simulink model "Cooperative_Quad_Rev01_4Agents_9"  (R2017b)
settings: Solver=ode45  StartTime=0.0  StopTime=120  RelTol=1e-3  EnableMultiTasking=on
InitFcn:
  | constant_Rev01_4Agents_9
values from neighbouring files (symbols this model uses):
  alpha = 0.1    [constant_Rev01_4Agents_9.m]
  alpha1 = 0.01    [constant_Rev01_4Agents_9.m]
  AN = [     0 1 0 0 ... (first row only)    [constant_Rev01_4Agents_9.m]
  B = 1e0*eye(n)    [constant_Rev01_4Agents_9.m]
  BBT_inv = ((B'*B)^(-1))*B'    [constant_Rev01_4Agents_9.m]
  BN = [     1 0 0 0 ... (first row only)    [constant_Rev01_4Agents_9.m]
  epsilon_struct = struct('data',epsilon_InitVal)    [constant_Rev01_4Agents_9.m]
  g = 9.81    [constant_Rev01_4Agents_9.m]
  gamma_0 = 1e+1*diag([1e-3*ones(6,1);1e-0*ones(6,1)])    [constant_Rev01_4Agents_9.m]
  gamma_1 = 1e+3*diag([1e-3*ones(6,1);1e0*ones(6,1)])    [constant_Rev01_4Agents_9.m]
  H = L + BN    [constant_Rev01_4Agents_9.m]
  J = 1.2416e-3 * diag([1 1 2],0)    [constant_Rev01_4Agents_9.m]
  k1 = 1    [constant_Rev01_4Agents_9.m]
  k2 = 1    [constant_Rev01_4Agents_9.m]
  Ka = 0.01    [constant_Rev01_4Agents_9.m]
  Kd = 0.01    [constant_Rev01_4Agents_9.m]
  Kf = 1e-5    (= 1e-05)    [constant_Rev01_4Agents_9.m]
  Ki = 1    [constant_Rev01_4Agents_9.m]
  Kt = 0.01 * Kf    (= 1e-07)    [constant_Rev01_4Agents_9.m]
  Lq = 0.2    [constant_Rev01_4Agents_9.m]
  M = 2    [constant_Rev01_4Agents_9.m]
  n = 12    [constant_Rev01_4Agents_9.m]
  N = 4    [constant_Rev01_4Agents_9.m]
  n0 = 3    [constant_Rev01_4Agents_9.m]
  Observer_Gain = 100    [constant_Rev01_4Agents_9.m]
  Observer_Gain1 = 10    [constant_Rev01_4Agents_9.m]
  Q = 1e-3*eye(n)    [constant_Rev01_4Agents_9.m]
  R = 1e-0*eye(n)    [constant_Rev01_4Agents_9.m]
  rho_0 = 1e+1    (= 10)    [constant_Rev01_4Agents_9.m]
  rho_1 = 1e-1    (= 0.1)    [constant_Rev01_4Agents_9.m]
  RM_1 = RM^(-1)    [constant_Rev01_4Agents_9.m]
  T_struct = struct('data',T_InitVal)    [constant_Rev01_4Agents_9.m]
  U_dot0_M = U_dot0_m*ones(n0,1)    [constant_Rev01_4Agents_9.m]
  Upsilon_M = Upsilon_m*ones(n0,1)    [constant_Rev01_4Agents_9.m]
undefined symbols (not defined in the file or in its folder): sigbuilder_block
(part 1 of 2)
settings Model: SimulationMode=rapid-accelerator  Creator=hp  LastModifiedBy=ali.safaei
settings DataIOCC: LimitDataPoints=on  SaveFormat=Array
settings OptimizationCC: LifeSpan=inf
settings DebuggingCC: UnderspecifiedInitializationDetection=Classic  MergeDetectMultiDrivingBlocksExec=none  SFUnexpectedBacktrackingDiag=warning  SFNoUnconditionalDefaultTransitionDiag=warning  SFExecutionAtInitializationDiag=none
settings HardwareCC: ProdBitPerPointer=32  ProdBitPerSizeT=32  ProdBitPerPtrDiffT=32  ProdLargestAtomicFloat=None  ProdIntDivRoundTo=Undefined  ProdEndianess=Unspecified  ProdWordSize=32  ProdHWDeviceType=32-bit Generic
settings ModelReferenceCC: PropagateSignalLabelsOutOfModel=off
settings CodeAppCC: StateflowObjectComments=on
settings GRTTargetCC: TargetLangStandard=C89/C90 (ANSI)  GeneratePreprocessorConditionals=Disable all
settings ConfigComp: CovMetricSettings=dw  CovHtmlReporting=on  CovSaveCumulativeToWorkspaceVar=on  CovSaveSingleToWorkspaceVar=on  CovExternalEMLEnable=off

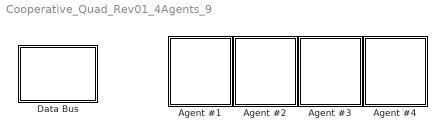
== system Cooperative_Quad_Rev01_4Agents_9 ==
  Agent #1 : Subsystem
  Agent #2 : Subsystem
  Agent #3 : Subsystem
  Agent #4 : Subsystem
  "Data Bus " : Subsystem

== system Cooperative_Quad_Rev01_4Agents_9/Agent #1 ==
  Agent # : Constant
  Controller interpreter : MATLAB Function  TreatAsAtomicUnit=on
  Decenteralized Cooperaive Controller #1 : Subsystem
  Plant #1 : Subsystem
  tag scope: x1=global
  wires:
  Decenteralized Cooperaive Controller #1/1(u1) -> Controller interpreter/1(U)
  Agent #/1 -> Decenteralized Cooperaive Controller #1/1(Agent #)
  Plant #1/1(X) -> [x1]
  Controller interpreter/1(u) -> Plant #1/1(U)

== system Cooperative_Quad_Rev01_4Agents_9/Agent #2 ==
  Agent # : Constant  Value=2
  Controller interpreter : MATLAB Function  TreatAsAtomicUnit=on
  Decenteralized Cooperaive Controller #2 : Subsystem
  Plant #2 : Subsystem
  tag scope: x2=global
  wires:
  Controller interpreter/1(u) -> Plant #2/1(U)
  Plant #2/1(X) -> [x2]
  Agent #/1 -> Decenteralized Cooperaive Controller #2/1(Agent #)
  Decenteralized Cooperaive Controller #2/1(u2) -> Controller interpreter/1(U)

== system Cooperative_Quad_Rev01_4Agents_9/Agent #3 ==
  Agent # : Constant  Value=3
  Controller interpreter : MATLAB Function  TreatAsAtomicUnit=on
  Decenteralized Cooperaive Controller #3 : Subsystem
  Plant #3 : Subsystem
  tag scope: x3=global
  wires:
  Decenteralized Cooperaive Controller #3/1(u3) -> Controller interpreter/1(U)
  Agent #/1 -> Decenteralized Cooperaive Controller #3/1(Agent #)
  Plant #3/1(X) -> [x3]
  Controller interpreter/1(u) -> Plant #3/1(U)

== system Cooperative_Quad_Rev01_4Agents_9/Agent #4 ==
  Agent # : Constant  Value=4
  Controller interpreter : MATLAB Function  TreatAsAtomicUnit=on
  Decenteralized Cooperaive Controller #4 : Subsystem
  Plant #4 : Subsystem
  tag scope: x4=global
  wires:
  Controller interpreter/1(u) -> Plant #4/1(U)
  Plant #4/1(X) -> [x4]
  Agent #/1 -> Decenteralized Cooperaive Controller #4/1(Agent #)
  Decenteralized Cooperaive Controller #4/1(u4) -> Controller interpreter/1(U)

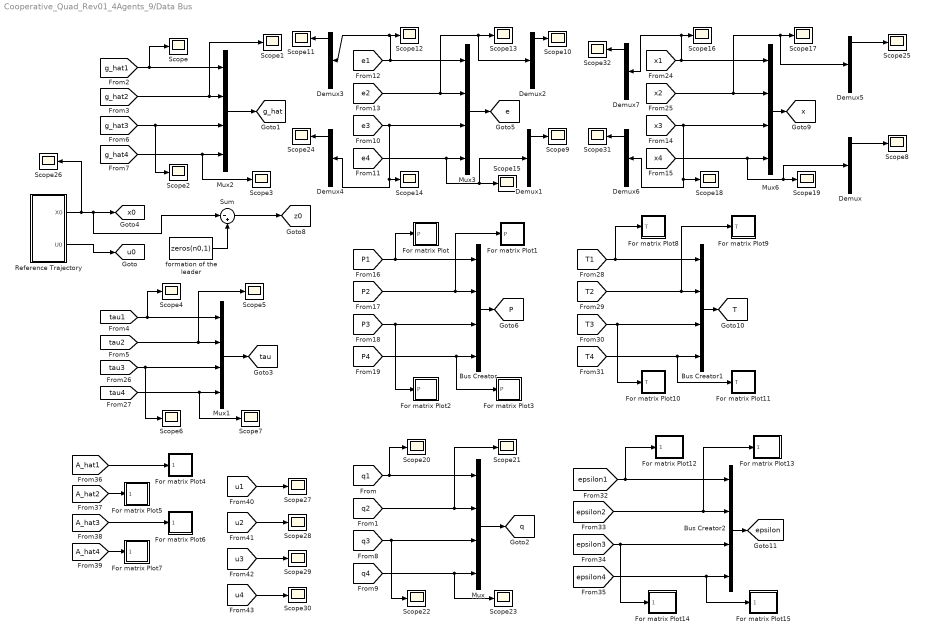
== system Cooperative_Quad_Rev01_4Agents_9/Data Bus  ==
  Bus Creator : BusCreator  Inputs=4  OutDataTypeStr=Bus: P_bus
  Bus Creator1 : BusCreator  Inputs=4  OutDataTypeStr=Bus: T_bus
  Bus Creator2 : BusCreator  Inputs=4  OutDataTypeStr=Bus: epsilon_bus
  Demux{,1..7} (8 alike) : Demux
  For matrix Plot : Subsystem
  For matrix Plot1 : Subsystem
  For matrix Plot10 : Subsystem
  For matrix Plot11 : Subsystem
  For matrix Plot12 : Subsystem
  For matrix Plot13 : Subsystem
  For matrix Plot14 : Subsystem
  For matrix Plot15 : Subsystem
  For matrix Plot2 : Subsystem
  For matrix Plot3 : Subsystem
  For matrix Plot4 : Subsystem
  For matrix Plot5 : Subsystem
  For matrix Plot6 : Subsystem
  For matrix Plot7 : Subsystem
  For matrix Plot8 : Subsystem
  For matrix Plot9 : Subsystem
  Mux{,1..3,6} (5 alike) : Mux
  Reference Trajectory : Subsystem
  Scope{,1..32} (33 alike) : Scope
  Sum : Sum  Inputs=|-+
  formation of the leader : Constant  Value=zeros(n0,1)
  tag scope: P=global, T=global, e=global, epsilon=global, g_hat=global, q=global, tau=global, u0=global, x0=global, x=global, z0=global
  wires:
  [q2] -> Scope21/1, Mux/2
  [tau1] -> Scope4/1, Mux1/1
  [tau2] -> Scope5/1, Mux1/2
  Mux1/1 -> [tau]
  [q1] -> Scope20/1, Mux/1
  Reference Trajectory/2(U0) -> [u0]
  [g_hat2] -> Mux2/2, Scope1/1
  Mux2/1 -> [g_hat]
  [g_hat1] -> Mux2/1, Scope/1
  Mux/1 -> [q]
  Reference Trajectory/1(X0) -> [x0], Sum/1, Scope26/1
  [e2] -> Demux2/1, Scope13/1, Mux3/2
  [e1] -> Scope12/1, Demux3/1, Mux3/1
  Mux3/1 -> [e]
  [P2] -> For matrix Plot1/1(P), Bus Creator/2
  [P1] -> For matrix Plot/1(P), Bus Creator/1
  Bus Creator/1 -> [P]
  Sum/1 -> [z0]
  formation of the leader/1 -> Sum/2
  [x1] -> Scope16/1, Demux7/1, Mux6/1
  Mux6/1 -> [x]
  [g_hat3] -> Scope2/1, Mux2/3
  [g_hat4] -> Scope3/1, Mux2/4
  [q4] -> Scope23/1, Mux/4
  [q3] -> Scope22/1, Mux/3
  [e3] -> Demux4/1, Scope14/1, Mux3/3
  [e4] -> Demux1/1, Scope15/1, Mux3/4
  [x3] -> Demux6/1, Scope18/1, Mux6/3
  [x4] -> Demux/1, Scope19/1, Mux6/4
  [P3] -> For matrix Plot2/1(P), Bus Creator/3
  [P4] -> For matrix Plot3/1(P), Bus Creator/4
  [tau3] -> Scope6/1, Mux1/3
  [tau4] -> Scope7/1, Mux1/4
  [T2] -> For matrix Plot9/1(T), Bus Creator1/2
  [T1] -> For matrix Plot8/1(T), Bus Creator1/1
  Bus Creator1/1 -> [T]
  [T3] -> For matrix Plot10/1(T), Bus Creator1/3
  [T4] -> For matrix Plot11/1(T), Bus Creator1/4
  [epsilon2] -> For matrix Plot13/1(epsilon), Bus Creator2/2
  [epsilon1] -> For matrix Plot12/1(epsilon), Bus Creator2/1
  Bus Creator2/1 -> [epsilon]
  [epsilon3] -> For matrix Plot14/1(epsilon), Bus Creator2/3
  [epsilon4] -> For matrix Plot15/1(epsilon), Bus Creator2/4
  [A_hat2] -> For matrix Plot5/1(A_hat)
  [A_hat1] -> For matrix Plot4/1(A_hat)
  [A_hat3] -> For matrix Plot6/1(A_hat)
  [A_hat4] -> For matrix Plot7/1(A_hat)
  [u2] -> Scope28/1
  [u1] -> Scope27/1
  [u4] -> Scope30/1
  [u3] -> Scope29/1
  Demux/1 -> Scope8/1
  Demux1/1 -> Scope9/1
  Demux2/1 -> Scope10/1
  Demux3/1 -> Scope11/1
  Demux4/1 -> Scope24/1
  [x2] -> Demux5/1, Scope17/1, Mux6/2
  Demux5/1 -> Scope25/1
  Demux6/1 -> Scope31/1
  Demux7/1 -> Scope32/1

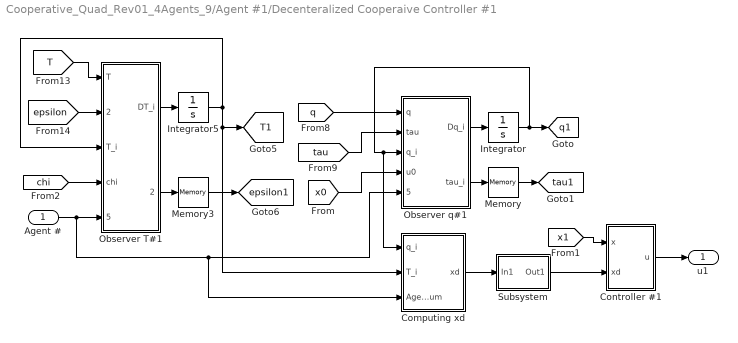
== system Cooperative_Quad_Rev01_4Agents_9/Agent #1/Decenteralized Cooperaive Controller #1 ==
  Agent # : Inport
  "Computing xd " : MATLAB Function  TreatAsAtomicUnit=on
  Controller #1 : Subsystem
  Integrator : Integrator  InitialCondition=zeros(n0,1)
  Integrator5 : Integrator  InitialCondition=zeros(N+1,n0)
  Memory : Memory  InitialCondition=zeros(n0,1)
  Memory3 : Memory  InitialCondition=zeros(N+1,n0)
  Observer T#1 : MATLAB Function  TreatAsAtomicUnit=on
  Observer q#1 : MATLAB Function  TreatAsAtomicUnit=on
  Subsystem : Subsystem
  u1 : Outport
  tag scope: T1=global, epsilon1=global, q1=global, tau1=global
  wires:
  [x0] -> Observer q#1/4(u0)
  [epsilon] -> Observer T#1/2(epsilon)
  [T] -> Observer T#1/1(T)
  Memory3/1 -> [epsilon1]
  Observer T#1/2(epsilon_i) -> Memory3/1
  Integrator5/1 -> [T1], "Computing xd "/2(T_i), Observer T#1/3(T_i)
  Observer T#1/1(DT_i) -> Integrator5/1
  [tau] -> Observer q#1/2(tau)
  [q] -> Observer q#1/1(q)
  Integrator/1 -> [q1], Observer q#1/3(q_i), "Computing xd "/1(q_i)
  Observer q#1/2(tau_i) -> Memory/1
  Observer q#1/1(Dq_i) -> Integrator/1
  Agent #/1 -> Observer T#1/5(Agent_Num), "Computing xd "/3(Agent_Num), Observer q#1/5(Agent_Num)
  Memory/1 -> [tau1]
  Controller #1/1(u) -> u1/1
  [x1] -> Controller #1/1(x)
  "Computing xd "/1(xd) -> Subsystem/1(In1)
  Subsystem/1(Out1) -> Controller #1/2(xd)
  [chi] -> Observer T#1/4(chi)

== system Cooperative_Quad_Rev01_4Agents_9/Agent #1/Plant #1 ==
  U : Inport
  Clock : Clock
  Demux1 : Demux
  Integrator : Integrator  InitialCondition=zeros(n,1)
  MATLAB Function : MATLAB Function  TreatAsAtomicUnit=on
  X : Outport
  wires:
  MATLAB Function/1(DX) -> Integrator/1
  Integrator/1 -> MATLAB Function/1(X), X/1
  Demux1/1 -> MATLAB Function/2(u1)
  Demux1/2 -> MATLAB Function/3(u2)
  Demux1/3 -> MATLAB Function/4(u3)
  Demux1/4 -> MATLAB Function/5(u4)
  U/1 -> Demux1/1
  Clock/1 -> MATLAB Function/6(t)

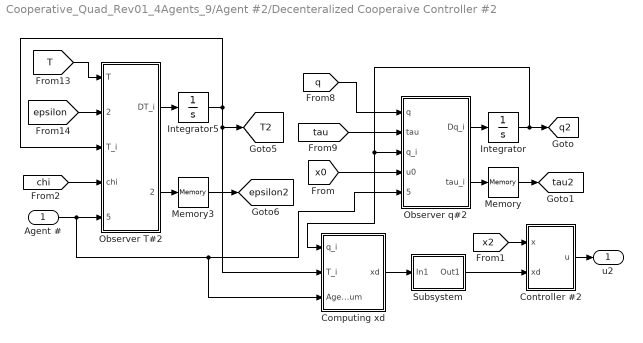
== system Cooperative_Quad_Rev01_4Agents_9/Agent #2/Decenteralized Cooperaive Controller #2 ==
  Agent # : Inport
  "Computing xd " : MATLAB Function  TreatAsAtomicUnit=on
  Controller #2 : Subsystem
  Integrator : Integrator  InitialCondition=zeros(n0,1)
  Integrator5 : Integrator  InitialCondition=zeros(N+1,n0)
  Memory : Memory  InitialCondition=zeros(n0,1)
  Memory3 : Memory  InitialCondition=zeros(N+1,n0)
  Observer T#2 : MATLAB Function  TreatAsAtomicUnit=on
  Observer q#2 : MATLAB Function  TreatAsAtomicUnit=on
  Subsystem : Subsystem
  u2 : Outport
  tag scope: T2=global, epsilon2=global, q2=global, tau2=global
  wires:
  [x2] -> Controller #2/1(x)
  Controller #2/1(u) -> u2/1
  Memory/1 -> [tau2]
  Agent #/1 -> Observer T#2/5(Agent_Num), Observer q#2/5(Agent_Num), "Computing xd "/3(Agent_Num)
  Observer q#2/1(Dq_i) -> Integrator/1
  Observer q#2/2(tau_i) -> Memory/1
  Integrator/1 -> Observer q#2/3(q_i), "Computing xd "/1(q_i), [q2]
  [q] -> Observer q#2/1(q)
  [tau] -> Observer q#2/2(tau)
  Observer T#2/1(DT_i) -> Integrator5/1
  Integrator5/1 -> Observer T#2/3(T_i), "Computing xd "/2(T_i), [T2]
  Observer T#2/2(epsilon_i) -> Memory3/1
  Memory3/1 -> [epsilon2]
  [T] -> Observer T#2/1(T)
  [epsilon] -> Observer T#2/2(epsilon)
  [x0] -> Observer q#2/4(u0)
  "Computing xd "/1(xd) -> Subsystem/1(In1)
  Subsystem/1(Out1) -> Controller #2/2(xd)
  [chi] -> Observer T#2/4(chi)

== system Cooperative_Quad_Rev01_4Agents_9/Agent #2/Plant #2 ==
  U : Inport
  Clock : Clock
  Demux1 : Demux
  Integrator : Integrator  InitialCondition=zeros(n,1)
  MATLAB Function : MATLAB Function  TreatAsAtomicUnit=on
  X : Outport
  wires:
  MATLAB Function/1(DX) -> Integrator/1
  Integrator/1 -> MATLAB Function/1(X), X/1
  Demux1/1 -> MATLAB Function/2(u1)
  Demux1/2 -> MATLAB Function/3(u2)
  Demux1/3 -> MATLAB Function/4(u3)
  Demux1/4 -> MATLAB Function/5(u4)
  U/1 -> Demux1/1
  Clock/1 -> MATLAB Function/6(t)

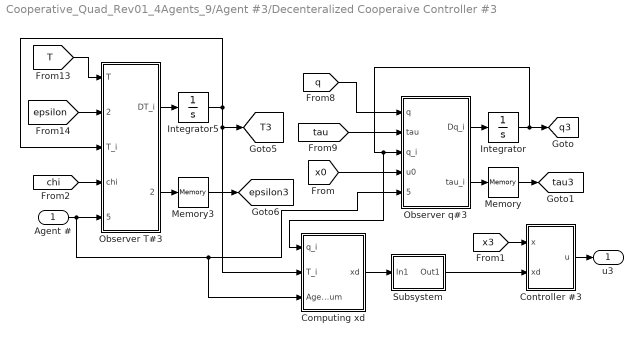
== system Cooperative_Quad_Rev01_4Agents_9/Agent #3/Decenteralized Cooperaive Controller #3 ==
  Agent # : Inport
  "Computing xd " : MATLAB Function  TreatAsAtomicUnit=on
  Controller #3 : Subsystem
  Integrator : Integrator  InitialCondition=zeros(n0,1)
  Integrator5 : Integrator  InitialCondition=zeros(N+1,n0)
  Memory : Memory  InitialCondition=zeros(n0,1)
  Memory3 : Memory  InitialCondition=zeros(N+1,n0)
  Observer T#3 : MATLAB Function  TreatAsAtomicUnit=on
  Observer q#3 : MATLAB Function  TreatAsAtomicUnit=on
  Subsystem : Subsystem
  u3 : Outport
  tag scope: T3=global, epsilon3=global, q3=global, tau3=global
  wires:
  [x0] -> Observer q#3/4(u0)
  [epsilon] -> Observer T#3/2(epsilon)
  [T] -> Observer T#3/1(T)
  Memory3/1 -> [epsilon3]
  Observer T#3/2(epsilon_i) -> Memory3/1
  Integrator5/1 -> [T3], "Computing xd "/2(T_i), Observer T#3/3(T_i)
  Observer T#3/1(DT_i) -> Integrator5/1
  [tau] -> Observer q#3/2(tau)
  [q] -> Observer q#3/1(q)
  Integrator/1 -> [q3], Observer q#3/3(q_i), "Computing xd "/1(q_i)
  Observer q#3/2(tau_i) -> Memory/1
  Observer q#3/1(Dq_i) -> Integrator/1
  Agent #/1 -> Observer T#3/5(Agent_Num), "Computing xd "/3(Agent_Num), Observer q#3/5(Agent_Num)
  Memory/1 -> [tau3]
  Controller #3/1(u) -> u3/1
  [x3] -> Controller #3/1(x)
  "Computing xd "/1(xd) -> Subsystem/1(In1)
  Subsystem/1(Out1) -> Controller #3/2(xd)
  [chi] -> Observer T#3/4(chi)

== system Cooperative_Quad_Rev01_4Agents_9/Agent #3/Plant #3 ==
  U : Inport
  Clock : Clock
  Demux1 : Demux
  Integrator : Integrator  InitialCondition=zeros(n,1)
  MATLAB Function : MATLAB Function  TreatAsAtomicUnit=on
  X : Outport
  wires:
  MATLAB Function/1(DX) -> Integrator/1
  Integrator/1 -> MATLAB Function/1(X), X/1
  Demux1/1 -> MATLAB Function/2(u1)
  Demux1/2 -> MATLAB Function/3(u2)
  Demux1/3 -> MATLAB Function/4(u3)
  Demux1/4 -> MATLAB Function/5(u4)
  U/1 -> Demux1/1
  Clock/1 -> MATLAB Function/6(t)

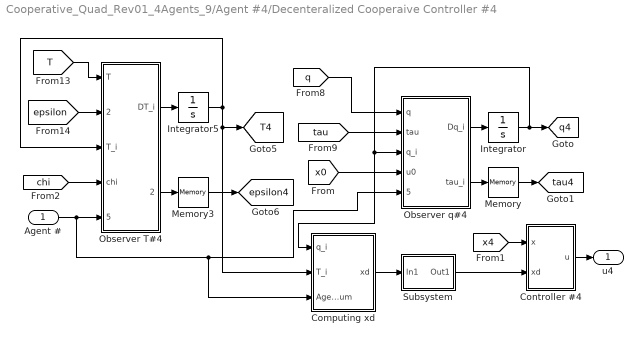
== system Cooperative_Quad_Rev01_4Agents_9/Agent #4/Decenteralized Cooperaive Controller #4 ==
  Agent # : Inport
  "Computing xd " : MATLAB Function  TreatAsAtomicUnit=on
  Controller #4 : Subsystem
  Integrator : Integrator  InitialCondition=zeros(n0,1)
  Integrator5 : Integrator  InitialCondition=zeros(N+1,n0)
  Memory : Memory  InitialCondition=zeros(n0,1)
  Memory3 : Memory  InitialCondition=zeros(N+1,n0)
  Observer T#4 : MATLAB Function  TreatAsAtomicUnit=on
  Observer q#4 : MATLAB Function  TreatAsAtomicUnit=on
  Subsystem : Subsystem
  u4 : Outport
  tag scope: T4=global, epsilon4=global, q4=global, tau4=global
  wires:
  [x4] -> Controller #4/1(x)
  Controller #4/1(u) -> u4/1
  Memory/1 -> [tau4]
  Agent #/1 -> Observer T#4/5(Agent_Num), Observer q#4/5(Agent_Num), "Computing xd "/3(Agent_Num)
  Observer q#4/1(Dq_i) -> Integrator/1
  Observer q#4/2(tau_i) -> Memory/1
  Integrator/1 -> Observer q#4/3(q_i), "Computing xd "/1(q_i), [q4]
  [q] -> Observer q#4/1(q)
  [tau] -> Observer q#4/2(tau)
  Observer T#4/1(DT_i) -> Integrator5/1
  Integrator5/1 -> Observer T#4/3(T_i), "Computing xd "/2(T_i), [T4]
  Observer T#4/2(epsilon_i) -> Memory3/1
  Memory3/1 -> [epsilon4]
  [T] -> Observer T#4/1(T)
  [epsilon] -> Observer T#4/2(epsilon)
  [x0] -> Observer q#4/4(u0)
  "Computing xd "/1(xd) -> Subsystem/1(In1)
  Subsystem/1(Out1) -> Controller #4/2(xd)
  [chi] -> Observer T#4/4(chi)

== system Cooperative_Quad_Rev01_4Agents_9/Agent #4/Plant #4 ==
  U : Inport
  Clock : Clock
  Demux1 : Demux
  Integrator : Integrator  InitialCondition=zeros(n,1)
  MATLAB Function : MATLAB Function  TreatAsAtomicUnit=on
  X : Outport
  wires:
  MATLAB Function/1(DX) -> Integrator/1
  Integrator/1 -> MATLAB Function/1(X), X/1
  Demux1/1 -> MATLAB Function/2(u1)
  Demux1/2 -> MATLAB Function/3(u2)
  Demux1/3 -> MATLAB Function/4(u3)
  Demux1/4 -> MATLAB Function/5(u4)
  U/1 -> Demux1/1
  Clock/1 -> MATLAB Function/6(t)

== system Cooperative_Quad_Rev01_4Agents_9/Data Bus /For matrix Plot ==
  P : Inport
  MATLAB Function : MATLAB Function  TreatAsAtomicUnit=on
  Scope24 : Scope
  To Workspace : ToWorkspace  VariableName=P1  SaveFormat=Structure With Time  SampleTime=-1
  wires:
  P/1 -> MATLAB Function/1(u)
  MATLAB Function/1(y) -> Scope24/1, To Workspace/1

== system Cooperative_Quad_Rev01_4Agents_9/Data Bus /For matrix Plot1 ==
  P : Inport
  MATLAB Function : MATLAB Function  TreatAsAtomicUnit=on
  Scope24 : Scope
  To Workspace : ToWorkspace  VariableName=P2  SaveFormat=Structure With Time  SampleTime=-1
  wires:
  MATLAB Function/1(y) -> Scope24/1, To Workspace/1
  P/1 -> MATLAB Function/1(u)

== system Cooperative_Quad_Rev01_4Agents_9/Data Bus /For matrix Plot10 ==
  T : Inport
  MATLAB Function : MATLAB Function  TreatAsAtomicUnit=on
  Scope24 : Scope
  To Workspace : ToWorkspace  VariableName=T3  SaveFormat=Structure With Time  SampleTime=-1
  wires:
  T/1 -> MATLAB Function/1(u)
  MATLAB Function/1(y) -> Scope24/1, To Workspace/1

== system Cooperative_Quad_Rev01_4Agents_9/Data Bus /For matrix Plot11 ==
  T : Inport
  MATLAB Function : MATLAB Function  TreatAsAtomicUnit=on
  Scope24 : Scope
  To Workspace : ToWorkspace  VariableName=T4  SaveFormat=Structure With Time  SampleTime=-1
  wires:
  MATLAB Function/1(y) -> Scope24/1, To Workspace/1
  T/1 -> MATLAB Function/1(u)

== system Cooperative_Quad_Rev01_4Agents_9/Data Bus /For matrix Plot12 ==
  epsilon : Inport
  MATLAB Function : MATLAB Function  TreatAsAtomicUnit=on
  Scope24 : Scope
  To Workspace : ToWorkspace  VariableName=epsilon1  SaveFormat=Structure With Time  SampleTime=-1
  wires:
  epsilon/1 -> MATLAB Function/1(u)
  MATLAB Function/1(y) -> Scope24/1, To Workspace/1

== system Cooperative_Quad_Rev01_4Agents_9/Data Bus /For matrix Plot13 ==
  epsilon : Inport
  MATLAB Function : MATLAB Function  TreatAsAtomicUnit=on
  Scope24 : Scope
  To Workspace : ToWorkspace  VariableName=epsilon2  SaveFormat=Structure With Time  SampleTime=-1
  wires:
  MATLAB Function/1(y) -> Scope24/1, To Workspace/1
  epsilon/1 -> MATLAB Function/1(u)

== system Cooperative_Quad_Rev01_4Agents_9/Data Bus /For matrix Plot14 ==
  epsilon : Inport
  MATLAB Function : MATLAB Function  TreatAsAtomicUnit=on
  Scope24 : Scope
  To Workspace : ToWorkspace  VariableName=epsilon3  SaveFormat=Structure With Time  SampleTime=-1
  wires:
  MATLAB Function/1(y) -> Scope24/1, To Workspace/1
  epsilon/1 -> MATLAB Function/1(u)

== system Cooperative_Quad_Rev01_4Agents_9/Data Bus /For matrix Plot15 ==
  epsilon : Inport
  MATLAB Function : MATLAB Function  TreatAsAtomicUnit=on
  Scope24 : Scope
  To Workspace : ToWorkspace  VariableName=epsilon4  SaveFormat=Structure With Time  SampleTime=-1
  wires:
  epsilon/1 -> MATLAB Function/1(u)
  MATLAB Function/1(y) -> Scope24/1, To Workspace/1

== system Cooperative_Quad_Rev01_4Agents_9/Data Bus /For matrix Plot2 ==
  P : Inport
  MATLAB Function : MATLAB Function  TreatAsAtomicUnit=on
  Scope24 : Scope
  To Workspace : ToWorkspace  VariableName=P3  SaveFormat=Structure With Time  SampleTime=-1
  wires:
  MATLAB Function/1(y) -> Scope24/1, To Workspace/1
  P/1 -> MATLAB Function/1(u)

== system Cooperative_Quad_Rev01_4Agents_9/Data Bus /For matrix Plot3 ==
  P : Inport
  MATLAB Function : MATLAB Function  TreatAsAtomicUnit=on
  Scope24 : Scope
  To Workspace : ToWorkspace  VariableName=P4  SaveFormat=Structure With Time  SampleTime=-1
  wires:
  P/1 -> MATLAB Function/1(u)
  MATLAB Function/1(y) -> Scope24/1, To Workspace/1

== system Cooperative_Quad_Rev01_4Agents_9/Data Bus /For matrix Plot4 ==
  A_hat : Inport
  MATLAB Function : MATLAB Function  TreatAsAtomicUnit=on
  Scope24 : Scope
  To Workspace : ToWorkspace  VariableName=A_hat1  SaveFormat=Structure With Time  SampleTime=-1
  wires:
  MATLAB Function/1(y) -> Scope24/1, To Workspace/1
  A_hat/1 -> MATLAB Function/1(u)

== system Cooperative_Quad_Rev01_4Agents_9/Data Bus /For matrix Plot5 ==
  A_hat : Inport
  MATLAB Function : MATLAB Function  TreatAsAtomicUnit=on
  Scope24 : Scope
  To Workspace : ToWorkspace  VariableName=A_hat2  SaveFormat=Structure With Time  SampleTime=-1
  wires:
  A_hat/1 -> MATLAB Function/1(u)
  MATLAB Function/1(y) -> Scope24/1, To Workspace/1

== system Cooperative_Quad_Rev01_4Agents_9/Data Bus /For matrix Plot6 ==
  A_hat : Inport
  MATLAB Function : MATLAB Function  TreatAsAtomicUnit=on
  Scope24 : Scope
  To Workspace : ToWorkspace  VariableName=A_hat3  SaveFormat=Structure With Time  SampleTime=-1
  wires:
  MATLAB Function/1(y) -> Scope24/1, To Workspace/1
  A_hat/1 -> MATLAB Function/1(u)

== system Cooperative_Quad_Rev01_4Agents_9/Data Bus /For matrix Plot7 ==
  A_hat : Inport
  MATLAB Function : MATLAB Function  TreatAsAtomicUnit=on
  Scope24 : Scope
  To Workspace : ToWorkspace  VariableName=A_hat4  SaveFormat=Structure With Time  SampleTime=-1
  wires:
  A_hat/1 -> MATLAB Function/1(u)
  MATLAB Function/1(y) -> Scope24/1, To Workspace/1

== system Cooperative_Quad_Rev01_4Agents_9/Data Bus /For matrix Plot8 ==
  T : Inport
  MATLAB Function : MATLAB Function  TreatAsAtomicUnit=on
  Scope24 : Scope
  To Workspace : ToWorkspace  VariableName=T1  SaveFormat=Structure With Time  SampleTime=-1
  wires:
  MATLAB Function/1(y) -> Scope24/1, To Workspace/1
  T/1 -> MATLAB Function/1(u)

== system Cooperative_Quad_Rev01_4Agents_9/Data Bus /For matrix Plot9 ==
  T : Inport
  MATLAB Function : MATLAB Function  TreatAsAtomicUnit=on
  Scope24 : Scope
  To Workspace : ToWorkspace  VariableName=T2  SaveFormat=Structure With Time  SampleTime=-1
  wires:
  T/1 -> MATLAB Function/1(u)
  MATLAB Function/1(y) -> Scope24/1, To Workspace/1

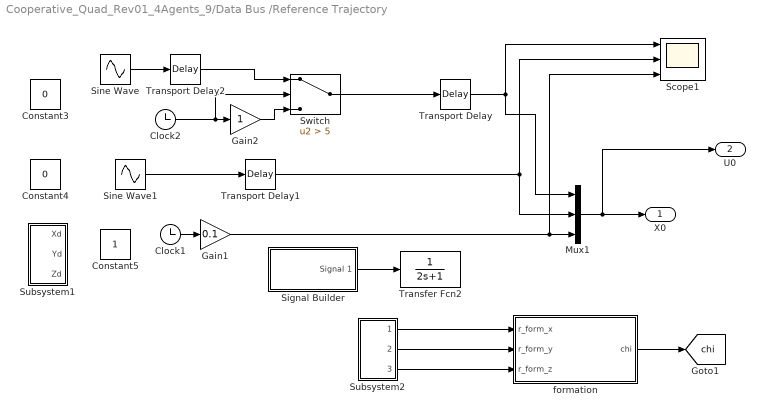
== system Cooperative_Quad_Rev01_4Agents_9/Data Bus /Reference Trajectory ==
  Clock1 : Clock
  Clock2 : Clock
  Constant3 : Constant  Value=0
  Constant4 : Constant  Value=0
  Constant5 : Constant
  Gain1 : Gain  Gain=0.1
  Gain2 : Gain
  Mux1 : Mux  Inputs=3
  Scope1 : Scope  NumInputPorts=3
  Signal Builder : Subsystem  Tag=STV Subsys  LoadFcn=sigbuilder_block('load');  StartFcn=sigbuilder_block('start');  StopFcn=sigbuilder_block('stop');  ClipboardFcn=sigbuilder_block('clipboard');  mask(Sigbuilder block){tuvar=[0:10]}
      mask help: Simulink:masks:SigbuilderBlock_MD
      mask init:
      | if ~strcmp(get_param(bdroot(gcbh),'SimulationStatus'),'stopped') tuvar = sigbuilder_block('maskInit'); end
      settings: CopyFcn=sigbuilder_block('copy');  DeleteFcn=sigbuilder_block('delete');  ModelCloseFcn=sigbuilder_block('modelClose');  PreSaveFcn=sigbuilder_block('preSave');  PauseFcn=sigbuilder_block('pause');  ContinueFcn=sigbuilder_block('continue');  NameChangeFcn=sigbuilder_block('namechange');  OpenFcn=sigbuilder_block('open',[437.25 117.75 550.5 394.5 ]);  CloseFcn=sigbuilder_block('close');
      mask Display: plot(0, 0, 100, 100,[2, 2, 32, 32, 2], [68, 8, 8, 68, 68],[32, 2], [38, 38], [32, 19, 2],[53, 60, 44], [32, 17, 17, 2],[16, 16, 31, 31]);txt = getActiveGroup(gcbh);text(2, 100, txt,'verticalAlignment', 'top');
  Sine Wave : Sin  Amplitude=5  Frequency=0.2  Phase=pi/2  SampleTime=0
  Sine Wave1 : Sin  Amplitude=5  Frequency=0.2  SampleTime=0
  Subsystem1 : Subsystem
  Subsystem2 : Subsystem
  Switch : Switch  Criteria=u2 > Threshold  Threshold=5
  Transfer Fcn2 : TransferFcn  Denominator=[2 1]
  Transport Delay : TransportDelay  DelayTime=5
  Transport Delay1 : TransportDelay  DelayTime=10
  Transport Delay2 : TransportDelay  DelayTime=5
  formation : MATLAB Function  TreatAsAtomicUnit=on
  X0 : Outport
  U0 : Outport  Port=2
  tag scope: chi=global
  wires:
  Clock1/1 -> Gain1/1
  Signal Builder/1(Signal 1) -> Transfer Fcn2/1
  Mux1/1 -> U0/1, X0/1
  Gain1/1 -> Scope1/3, Mux1/3
  Sine Wave1/1 -> Transport Delay1/1
  Transport Delay1/1 -> Mux1/2, Scope1/2
  Transport Delay/1 -> Mux1/1, Scope1/1
  formation/1(chi) -> [chi]
  Subsystem2/1(form_x) -> formation/1(r_form_x)
  Subsystem2/2(form_y) -> formation/2(r_form_y)
  Subsystem2/3(form_z) -> formation/3(r_form_z)
  Switch/1 -> Transport Delay/1
  Clock2/1 -> Switch/2, Gain2/1
  Sine Wave/1 -> Transport Delay2/1
  Gain2/1 -> Switch/3
  Transport Delay2/1 -> Switch/1

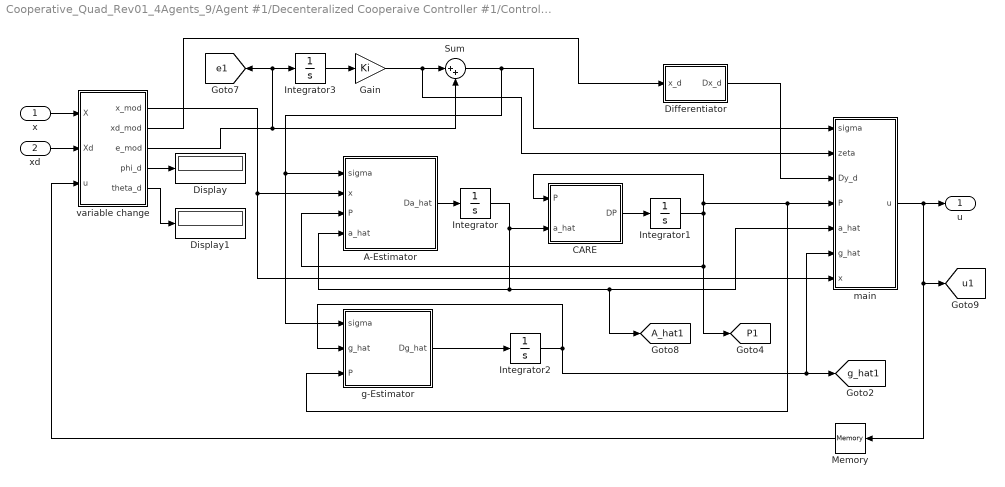
== system Cooperative_Quad_Rev01_4Agents_9/Agent #1/Decenteralized Cooperaive Controller #1/Controller #1 ==
  x : Inport
  xd : Inport  Port=2
  A-Estimator : MATLAB Function  TreatAsAtomicUnit=on
  CARE : MATLAB Function  TreatAsAtomicUnit=on
  Differentiator : Subsystem
  Display : Display
  Display1 : Display
  Gain : Gain  Gain=Ki
  Integrator : Integrator  InitialCondition=zeros(n)
  Integrator1 : Integrator  InitialCondition=eye(n)
  Integrator2 : Integrator  InitialCondition=zeros(n,1)
  Integrator3 : Integrator  InitialCondition=zeros(n,1)
  Memory : Memory  InitialCondition=zeros(n,1)
  Sum : Sum  Inputs=|++
  g-Estimator : MATLAB Function  TreatAsAtomicUnit=on
  main : MATLAB Function  TreatAsAtomicUnit=on
  variable change : MATLAB Function  TreatAsAtomicUnit=on
  u : Outport
  tag scope: A_hat1=global, P1=global, e1=global, g_hat1=global, u1=global
  wires:
  xd/1 -> variable change/2(Xd)
  x/1 -> variable change/1(X)
  Integrator/1 -> A-Estimator/4(a_hat), [A_hat1], main/5(a_hat), CARE/2(a_hat)
  Integrator1/1 -> main/4(P), g-Estimator/3(P), CARE/1(P), [P1], A-Estimator/3(P)
  Sum/1 -> A-Estimator/1(sigma), g-Estimator/1(sigma), main/1(sigma)
  Differentiator/1(Dx_d) -> main/3(Dy_d)
  variable change/2(xd_mod) -> Differentiator/1(x_d)
  A-Estimator/1(Da_hat) -> Integrator/1
  variable change/1(x_mod) -> A-Estimator/2(x), main/7(x)
  Integrator3/1 -> Gain/1
  variable change/3(e_mod) -> [e1], Integrator3/1, Sum/2
  Integrator2/1 -> g-Estimator/2(g_hat), [g_hat1], main/6(g_hat)
  g-Estimator/1(Dg_hat) -> Integrator2/1
  Gain/1 -> main/2(zeta), Sum/1
  Memory/1 -> variable change/3(u)
  main/1(u) -> [u1], Memory/1, u/1
  variable change/4(phi_d) -> Display/1
  variable change/5(theta_d) -> Display1/1
  CARE/1(DP) -> Integrator1/1

== system Cooperative_Quad_Rev01_4Agents_9/Agent #1/Decenteralized Cooperaive Controller #1/Subsystem ==
  In1 : Inport
  Demux : Demux  Outputs=3
  Mux : Mux  Inputs=3
  Transport Delay1 : TransportDelay  DelayTime=5
  Transport Delay2 : TransportDelay  DelayTime=5
  Out1 : Outport
  wires:
  In1/1 -> Demux/1
  Demux/1 -> Transport Delay1/1
  Demux/2 -> Transport Delay2/1
  Mux/1 -> Out1/1
  Transport Delay2/1 -> Mux/2
  Transport Delay1/1 -> Mux/1
  Demux/3 -> Mux/3

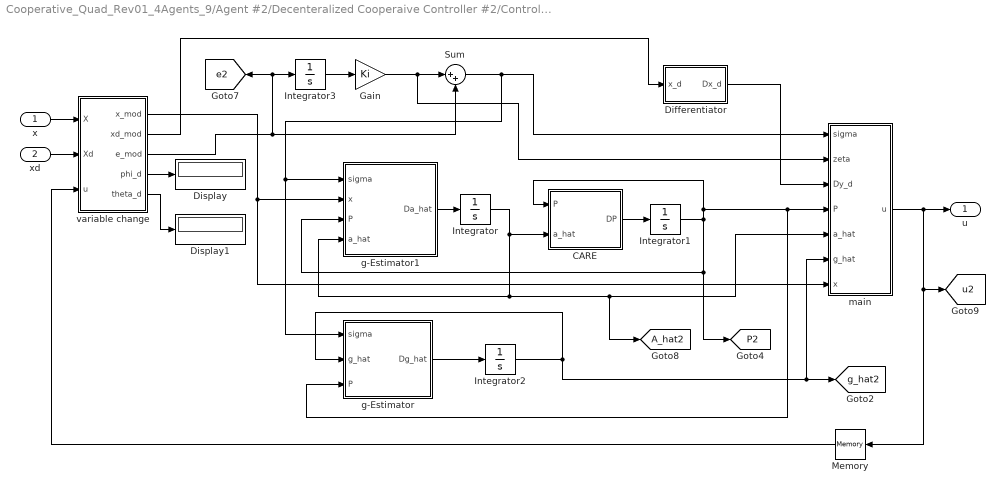
== system Cooperative_Quad_Rev01_4Agents_9/Agent #2/Decenteralized Cooperaive Controller #2/Controller #2 ==
  x : Inport
  xd : Inport  Port=2
  CARE : MATLAB Function  TreatAsAtomicUnit=on
  Differentiator : Subsystem
  Display : Display
  Display1 : Display
  Gain : Gain  Gain=Ki
  Integrator : Integrator  InitialCondition=zeros(n)
  Integrator1 : Integrator  InitialCondition=eye(n)
  Integrator2 : Integrator  InitialCondition=zeros(n,1)
  Integrator3 : Integrator  InitialCondition=zeros(n,1)
  Memory : Memory  InitialCondition=zeros(n,1)
  Sum : Sum  Inputs=|++
  g-Estimator : MATLAB Function  TreatAsAtomicUnit=on
  g-Estimator1 : MATLAB Function  TreatAsAtomicUnit=on
  main : MATLAB Function  TreatAsAtomicUnit=on
  variable change : MATLAB Function  TreatAsAtomicUnit=on
  u : Outport
  tag scope: A_hat2=global, P2=global, e2=global, g_hat2=global, u2=global
  wires:
  CARE/1(DP) -> Integrator1/1
  variable change/5(theta_d) -> Display1/1
  variable change/4(phi_d) -> Display/1
  main/1(u) -> Memory/1, [u2], u/1
  Memory/1 -> variable change/3(u)
  Gain/1 -> main/2(zeta), Sum/1
  g-Estimator/1(Dg_hat) -> Integrator2/1
  Integrator2/1 -> g-Estimator/2(g_hat), main/6(g_hat), [g_hat2]
  variable change/3(e_mod) -> Sum/2, Integrator3/1, [e2]
  Integrator3/1 -> Gain/1
  variable change/1(x_mod) -> main/7(x), g-Estimator1/2(x)
  g-Estimator1/1(Da_hat) -> Integrator/1
  variable change/2(xd_mod) -> Differentiator/1(x_d)
  Differentiator/1(Dx_d) -> main/3(Dy_d)
  Sum/1 -> main/1(sigma), g-Estimator/1(sigma), g-Estimator1/1(sigma)
  Integrator1/1 -> g-Estimator1/3(P), [P2], CARE/1(P), g-Estimator/3(P), main/4(P)
  Integrator/1 -> [A_hat2], main/5(a_hat), g-Estimator1/4(a_hat), CARE/2(a_hat)
  x/1 -> variable change/1(X)
  xd/1 -> variable change/2(Xd)

== system Cooperative_Quad_Rev01_4Agents_9/Agent #2/Decenteralized Cooperaive Controller #2/Subsystem ==
  In1 : Inport
  Demux : Demux  Outputs=3
  Mux : Mux  Inputs=3
  Transport Delay1 : TransportDelay  DelayTime=5
  Transport Delay2 : TransportDelay  DelayTime=5
  Out1 : Outport
  wires:
  In1/1 -> Demux/1
  Demux/1 -> Transport Delay1/1
  Demux/2 -> Transport Delay2/1
  Mux/1 -> Out1/1
  Transport Delay2/1 -> Mux/2
  Transport Delay1/1 -> Mux/1
  Demux/3 -> Mux/3

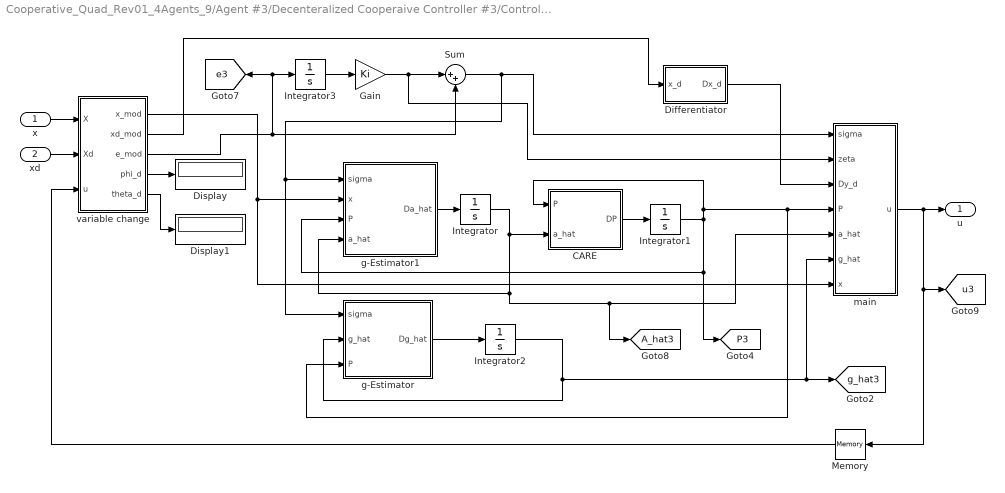
== system Cooperative_Quad_Rev01_4Agents_9/Agent #3/Decenteralized Cooperaive Controller #3/Controller #3 ==
  x : Inport
  xd : Inport  Port=2
  CARE : MATLAB Function  TreatAsAtomicUnit=on
  Differentiator : Subsystem
  Display : Display
  Display1 : Display
  Gain : Gain  Gain=Ki
  Integrator : Integrator  InitialCondition=zeros(n)
  Integrator1 : Integrator  InitialCondition=eye(n)
  Integrator2 : Integrator  InitialCondition=zeros(n,1)
  Integrator3 : Integrator  InitialCondition=zeros(n,1)
  Memory : Memory  InitialCondition=zeros(n,1)
  Sum : Sum  Inputs=|++
  g-Estimator : MATLAB Function  TreatAsAtomicUnit=on
  g-Estimator1 : MATLAB Function  TreatAsAtomicUnit=on
  main : MATLAB Function  TreatAsAtomicUnit=on
  variable change : MATLAB Function  TreatAsAtomicUnit=on
  u : Outport
  tag scope: A_hat3=global, P3=global, e3=global, g_hat3=global, u3=global
  wires:
  xd/1 -> variable change/2(Xd)
  x/1 -> variable change/1(X)
  Integrator/1 -> g-Estimator1/4(a_hat), [A_hat3], main/5(a_hat), CARE/2(a_hat)
  Integrator1/1 -> main/4(P), g-Estimator/3(P), CARE/1(P), [P3], g-Estimator1/3(P)
  Sum/1 -> g-Estimator1/1(sigma), g-Estimator/1(sigma), main/1(sigma)
  Differentiator/1(Dx_d) -> main/3(Dy_d)
  variable change/2(xd_mod) -> Differentiator/1(x_d)
  g-Estimator1/1(Da_hat) -> Integrator/1
  variable change/1(x_mod) -> g-Estimator1/2(x), main/7(x)
  Integrator3/1 -> Gain/1
  variable change/3(e_mod) -> [e3], Integrator3/1, Sum/2
  Integrator2/1 -> [g_hat3], main/6(g_hat), g-Estimator/2(g_hat)
  g-Estimator/1(Dg_hat) -> Integrator2/1
  Gain/1 -> main/2(zeta), Sum/1
  Memory/1 -> variable change/3(u)
  main/1(u) -> [u3], Memory/1, u/1
  variable change/4(phi_d) -> Display/1
  variable change/5(theta_d) -> Display1/1
  CARE/1(DP) -> Integrator1/1

== system Cooperative_Quad_Rev01_4Agents_9/Agent #3/Decenteralized Cooperaive Controller #3/Subsystem ==
  In1 : Inport
  Demux : Demux  Outputs=3
  Mux : Mux  Inputs=3
  Transport Delay1 : TransportDelay  DelayTime=5
  Transport Delay2 : TransportDelay  DelayTime=5
  Out1 : Outport
  wires:
  In1/1 -> Demux/1
  Demux/1 -> Transport Delay1/1
  Demux/2 -> Transport Delay2/1
  Mux/1 -> Out1/1
  Transport Delay2/1 -> Mux/2
  Transport Delay1/1 -> Mux/1
  Demux/3 -> Mux/3

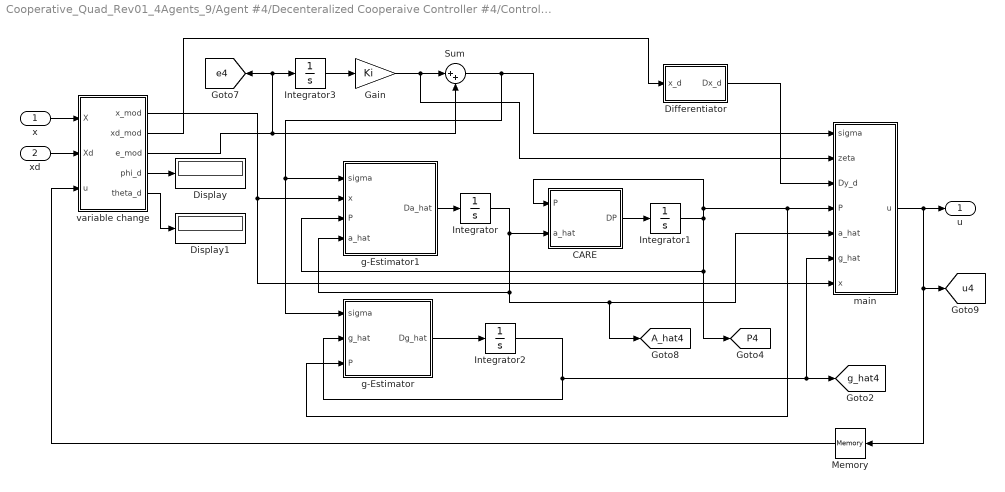
== system Cooperative_Quad_Rev01_4Agents_9/Agent #4/Decenteralized Cooperaive Controller #4/Controller #4 ==
  x : Inport
  xd : Inport  Port=2
  CARE : MATLAB Function  TreatAsAtomicUnit=on
  Differentiator : Subsystem
  Display : Display
  Display1 : Display
  Gain : Gain  Gain=Ki
  Integrator : Integrator  InitialCondition=zeros(n)
  Integrator1 : Integrator  InitialCondition=eye(n)
  Integrator2 : Integrator  InitialCondition=zeros(n,1)
  Integrator3 : Integrator  InitialCondition=zeros(n,1)
  Memory : Memory  InitialCondition=zeros(n,1)
  Sum : Sum  Inputs=|++
  g-Estimator : MATLAB Function  TreatAsAtomicUnit=on
  g-Estimator1 : MATLAB Function  TreatAsAtomicUnit=on
  main : MATLAB Function  TreatAsAtomicUnit=on
  variable change : MATLAB Function  TreatAsAtomicUnit=on
  u : Outport
  tag scope: A_hat4=global, P4=global, e4=global, g_hat4=global, u4=global
  wires:
  CARE/1(DP) -> Integrator1/1
  variable change/5(theta_d) -> Display1/1
  variable change/4(phi_d) -> Display/1
  main/1(u) -> u/1, Memory/1, [u4]
  Memory/1 -> variable change/3(u)
  Gain/1 -> main/2(zeta), Sum/1
  g-Estimator/1(Dg_hat) -> Integrator2/1
  Integrator2/1 -> g-Estimator/2(g_hat), main/6(g_hat), [g_hat4]
  variable change/3(e_mod) -> Sum/2, Integrator3/1, [e4]
  Integrator3/1 -> Gain/1
  variable change/1(x_mod) -> main/7(x), g-Estimator1/2(x)
  g-Estimator1/1(Da_hat) -> Integrator/1
  variable change/2(xd_mod) -> Differentiator/1(x_d)
  Differentiator/1(Dx_d) -> main/3(Dy_d)
  Sum/1 -> main/1(sigma), g-Estimator/1(sigma), g-Estimator1/1(sigma)
  Integrator1/1 -> g-Estimator1/3(P), [P4], CARE/1(P), g-Estimator/3(P), main/4(P)
  Integrator/1 -> g-Estimator1/4(a_hat), main/5(a_hat), [A_hat4], CARE/2(a_hat)
  x/1 -> variable change/1(X)
  xd/1 -> variable change/2(Xd)

== system Cooperative_Quad_Rev01_4Agents_9/Agent #4/Decenteralized Cooperaive Controller #4/Subsystem ==
  In1 : Inport
  Demux : Demux  Outputs=3
  Mux : Mux  Inputs=3
  Transport Delay1 : TransportDelay  DelayTime=5
  Transport Delay2 : TransportDelay  DelayTime=5
  Out1 : Outport
  wires:
  In1/1 -> Demux/1
  Demux/1 -> Transport Delay1/1
  Demux/2 -> Transport Delay2/1
  Mux/1 -> Out1/1
  Transport Delay2/1 -> Mux/2
  Transport Delay1/1 -> Mux/1
  Demux/3 -> Mux/3

== system Cooperative_Quad_Rev01_4Agents_9/Data Bus /Reference Trajectory/Signal Builder ==
  Demux : Demux  Tag=STV Demux  Outputs=1
  FromWs : FromWorkspace  Tag=STV FromWs  VariableName=tuvar  SampleTime=0
      SigBuilderData=|
      | common.afterFinalStr = 'Extrapolate'
      | common.sampleTime = 0
      | dataSet.timeRange = [0 100]
      | dataSet.name = 'Group 1'
      | sbobj.Groups.Name = 'Group 1'
      | sbobj.Groups.Signals.Name = 'Signal 1'
      | sbobj.Groups.Signals.XData = [0 20 20 50 50 100]
      | sbobj.Groups.Signals.YData = [0 0 2 2 0 0]
      | sbobj.Groups.TimeRange = [0 100]
  Signal 1 : Outport  Tag=STV Outport
  wires:
  Demux/1 -> Signal 1/1
  FromWs/1 -> Demux/1

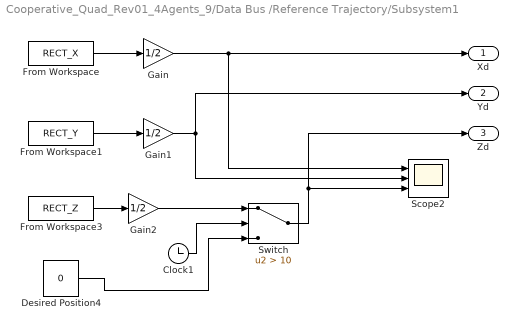
== system Cooperative_Quad_Rev01_4Agents_9/Data Bus /Reference Trajectory/Subsystem1 ==
  Clock1 : Clock
  Desired Position4 : Constant  Value=0  VectorParams1D=off
  From Workspace : FromWorkspace  VariableName=RECT_X  SampleTime=0
  From Workspace1 : FromWorkspace  VariableName=RECT_Y  SampleTime=0
  From Workspace3 : FromWorkspace  VariableName=RECT_Z  SampleTime=0
  Gain : Gain  Gain=1/2
  Gain1 : Gain  Gain=1/2
  Gain2 : Gain  Gain=1/2
  Scope2 : Scope  NumInputPorts=3
  Switch : Switch  Criteria=u2 > Threshold  Threshold=10
  Xd : Outport
  Yd : Outport  Port=2
  Zd : Outport  Port=3
  wires:
  From Workspace/1 -> Gain/1
  From Workspace1/1 -> Gain1/1
  Clock1/1 -> Switch/2
  Switch/1 -> Zd/1, Scope2/3
  From Workspace3/1 -> Gain2/1
  Desired Position4/1 -> Switch/3
  Gain/1 -> Xd/1, Scope2/1
  Gain1/1 -> Yd/1, Scope2/2
  Gain2/1 -> Switch/1

== system Cooperative_Quad_Rev01_4Agents_9/Data Bus /Reference Trajectory/Subsystem2 ==
  Clock1 : Clock
  Desired Position1 : Constant  Value=3  VectorParams1D=off
  Desired Position2 : Constant  VectorParams1D=off
  Desired Position3 : Constant  Value=-1  VectorParams1D=off
  Desired Position4 : Constant  Value=2  VectorParams1D=off
  Desired Position5 : Constant  Value=0.5  VectorParams1D=off
  Desired Position6 : Constant  Value=-0.5  VectorParams1D=off
  Switch : Switch  Criteria=u2 > Threshold  Threshold=50
  Switch1 : Switch  Criteria=u2 > Threshold  Threshold=50
  Switch2 : Switch  Criteria=u2 > Threshold  Threshold=50
  form_x : Outport
  form_y : Outport  Port=2
  form_z : Outport  Port=3
  wires:
  Desired Position1/1 -> Switch/1
  Switch1/1 -> form_y/1
  Switch2/1 -> form_x/1
  Desired Position4/1 -> Switch/3
  Switch/1 -> form_z/1
  Clock1/1 -> Switch1/2, Switch2/2, Switch/2
  Desired Position2/1 -> Switch1/1
  Desired Position3/1 -> Switch1/3
  Desired Position6/1 -> Switch2/3
  Desired Position5/1 -> Switch2/1

== system Cooperative_Quad_Rev01_4Agents_9/Agent #1/Decenteralized Cooperaive Controller #1/Controller #1/Differentiator ==
  x_d : Inport
  Integrator : Integrator  InitialCondition=zeros(n,1)
  Integrator1 : Integrator  InitialCondition=zeros(n,1)
  Sliding differentiator : MATLAB Function  TreatAsAtomicUnit=on
  Sliding differentiator1 : MATLAB Function  TreatAsAtomicUnit=on
  Sum : Sum  Inputs=|-+
  Dx_d : Outport
  wires:
  Sliding differentiator/1(u) -> Integrator1/1, Dx_d/1
  Sliding differentiator1/1(Du1) -> Integrator/1
  Integrator/1 -> Sliding differentiator/1(u1)
  x_d/1 -> Sum/1
  Sum/1 -> Sliding differentiator1/1(e), Sliding differentiator/2(e)
  Integrator1/1 -> Sum/2

== system Cooperative_Quad_Rev01_4Agents_9/Agent #2/Decenteralized Cooperaive Controller #2/Controller #2/Differentiator ==
  x_d : Inport
  Integrator : Integrator  InitialCondition=zeros(n,1)
  Integrator1 : Integrator  InitialCondition=zeros(n,1)
  Sliding differentiator : MATLAB Function  TreatAsAtomicUnit=on
  Sliding differentiator1 : MATLAB Function  TreatAsAtomicUnit=on
  Sum : Sum  Inputs=|-+
  Dx_d : Outport
  wires:
  Sliding differentiator/1(u) -> Integrator1/1, Dx_d/1
  Sliding differentiator1/1(Du1) -> Integrator/1
  Integrator/1 -> Sliding differentiator/1(u1)
  x_d/1 -> Sum/1
  Sum/1 -> Sliding differentiator1/1(e), Sliding differentiator/2(e)
  Integrator1/1 -> Sum/2

== system Cooperative_Quad_Rev01_4Agents_9/Agent #3/Decenteralized Cooperaive Controller #3/Controller #3/Differentiator ==
  x_d : Inport
  Integrator : Integrator  InitialCondition=zeros(n,1)
  Integrator1 : Integrator  InitialCondition=zeros(n,1)
  Sliding differentiator : MATLAB Function  TreatAsAtomicUnit=on
  Sliding differentiator1 : MATLAB Function  TreatAsAtomicUnit=on
  Sum : Sum  Inputs=|-+
  Dx_d : Outport
  wires:
  Sliding differentiator/1(u) -> Integrator1/1, Dx_d/1
  Sliding differentiator1/1(Du1) -> Integrator/1
  Integrator/1 -> Sliding differentiator/1(u1)
  x_d/1 -> Sum/1
  Sum/1 -> Sliding differentiator1/1(e), Sliding differentiator/2(e)
  Integrator1/1 -> Sum/2

== system Cooperative_Quad_Rev01_4Agents_9/Agent #4/Decenteralized Cooperaive Controller #4/Controller #4/Differentiator ==
  x_d : Inport
  Integrator : Integrator  InitialCondition=zeros(n,1)
  Integrator1 : Integrator  InitialCondition=zeros(n,1)
  Sliding differentiator : MATLAB Function  TreatAsAtomicUnit=on
  Sliding differentiator1 : MATLAB Function  TreatAsAtomicUnit=on
  Sum : Sum  Inputs=|-+
  Dx_d : Outport
  wires:
  Sliding differentiator/1(u) -> Integrator1/1, Dx_d/1
  Sliding differentiator1/1(Du1) -> Integrator/1
  Integrator/1 -> Sliding differentiator/1(u1)
  x_d/1 -> Sum/1
  Sum/1 -> Sliding differentiator1/1(e), Sliding differentiator/2(e)
  Integrator1/1 -> Sum/2

== matlab function Cooperative_Quad_Rev01_4Agents_9/Agent #1/Controller interpreter ==
  data: u output; U input; RM_1 parameter; n0 parameter; n parameter
function u = fcn(U,RM_1,n0,n)

y0 = sqrt((U(7)^2)+(U(8)^2)+(U(9)^2));
y1 = U(10);
y2 = U(11);
y3 = U(12);

Y = [y0;y1;y2;y3];

u = RM_1*Y;

for i=1:4
    u(i) = sqrt(abs(u(i)));
end

end

== matlab function Cooperative_Quad_Rev01_4Agents_9/Agent #1/Decenteralized Cooperaive Controller #1/Computing xd  ==
  data: q_i input; T_i input; xd output; Agent_Num input
function xd = fcn(q_i,T_i,Agent_Num)

xd = q_i + T_i(1,:)' + T_i(Agent_Num+1,:)';

end

== matlab function Cooperative_Quad_Rev01_4Agents_9/Agent #2/Controller interpreter ==
  data: u output; U input; RM_1 parameter; n0 parameter; n parameter
function u = fcn(U,RM_1,n0,n)

y0 = sqrt((U(7)^2)+(U(8)^2)+(U(9)^2));
y1 = U(10);
y2 = U(11);
y3 = U(12);

Y = [y0;y1;y2;y3];

u = RM_1*Y;

for i=1:4
    u(i) = sqrt(abs(u(i)));
end

end

== matlab function Cooperative_Quad_Rev01_4Agents_9/Agent #2/Decenteralized Cooperaive Controller #2/Computing xd  ==
  data: q_i input; T_i input; xd output; Agent_Num input
function xd = fcn(q_i,T_i,Agent_Num)

xd = q_i + T_i(1,:)' + T_i(Agent_Num+1,:)';

end

== matlab function Cooperative_Quad_Rev01_4Agents_9/Agent #2/Decenteralized Cooperaive Controller #2/Controller #2/CARE ==
  data: P input; a_hat input; B parameter; R parameter; DP output; Q parameter
function DP = fcn(P,a_hat,B,R,Q)

DP = a_hat*P + P*a_hat' - P*B*R*B'*P + 2*Q;

end

== matlab function Cooperative_Quad_Rev01_4Agents_9/Agent #2/Decenteralized Cooperaive Controller #2/Controller #2/Differentiator/Sliding differentiator ==
  data: u output; u1 input; e input; k1 parameter; alpha1 parameter
function u = fcn(u1,e,k1,alpha1)

b=k1;

ABS = abs(e);
SGN = e ./ (ABS + alpha1);
u = u1 - b*(ABS.^0.5).*SGN;

end

== matlab function Cooperative_Quad_Rev01_4Agents_9/Agent #2/Decenteralized Cooperaive Controller #2/Controller #2/Differentiator/Sliding differentiator1 ==
  data: Du1 output; e input; k2 parameter; alpha1 parameter
function Du1 = fcn(e,k2,alpha1)

a=k2;

ABS = abs(e);
SGN = e ./ (ABS + alpha1);
Du1 = - a*SGN;

end

== matlab function Cooperative_Quad_Rev01_4Agents_9/Agent #2/Decenteralized Cooperaive Controller #2/Controller #2/g-Estimator ==
  data: sigma input; g_hat input; P input; rho_1 parameter; gamma_1 parameter; Dg_hat output
function Dg_hat = fcn(sigma,g_hat,P,rho_1,gamma_1)

Dg_hat = - gamma_1 * P * sigma - rho_1 * gamma_1 * g_hat;

end

== matlab function Cooperative_Quad_Rev01_4Agents_9/Agent #2/Decenteralized Cooperaive Controller #2/Controller #2/g-Estimator1 ==
  data: sigma input; x input; P input; rho_0 parameter; gamma_0 parameter; Da_hat output; a_hat input
function Da_hat = fcn(sigma,x,P,rho_0,gamma_0,a_hat)

DVa_hat = - gamma_0 * P * diag(sigma) * (x - sigma) - rho_0 * gamma_0 * diag(a_hat);

Da_hat = diag(DVa_hat);

end

== matlab function Cooperative_Quad_Rev01_4Agents_9/Agent #2/Decenteralized Cooperaive Controller #2/Controller #2/main ==
  data: sigma input; zeta input; u output; Dy_d input; R parameter; P input; a_hat input; B parameter; g_hat input; x input; Q parameter; BBT_inv parameter; n parameter; Ki parameter
function u = fcn(sigma,zeta,Dy_d,R,P,a_hat,B,g_hat,x,Q,BBT_inv,n,Ki)

u1 = (1/2) * R * B' * P * sigma;
u2 = BBT_inv * (Dy_d - a_hat*x + (Ki*eye(n) + 2*(((P)^(-1)*Q)) + a_hat)*sigma - g_hat - Ki*zeta) - (3/4) * R * B' * P * sigma;

u = u1 + u2;

end

== matlab function Cooperative_Quad_Rev01_4Agents_9/Agent #1/Decenteralized Cooperaive Controller #1/Observer T#1 ==
  data: T_struct parameter; T input; DT_i output; epsilon input; epsilon_struct parameter; H parameter; BN parameter; AN parameter; T_i input; chi input; Upsilon_M parameter; epsilon_i output; N parameter; n0 parameter; Agent_Num input; Observer_Gain1 parameter; alpha parameter
function [DT_i,epsilon_i] = fcn(T_struct,T,epsilon,epsilon_struct,H,BN,AN,T_i,chi,Upsilon_M,N,n0,...
    Agent_Num,Observer_Gain1,alpha)

T_struct(1).data = T.t1;
T_struct(2).data = T.t2;
T_struct(3).data = T.t3;
T_struct(4).data = T.t4;

epsilon_struct(1).data = epsilon.eps1;
epsilon_struct(2).data = epsilon.eps2;
epsilon_struct(3).data = epsilon.eps3;
epsilon_struct(4).data = epsilon.eps4;

epsilon_i = + BN(Agent_Num,Agent_Num)*(T_i - chi);
Sum2 = zeros(N+1,n0);
for i=1:N
    epsilon_i = epsilon_i + ( AN(Agent_Num,i) * (T_i - T_struct(i).data) );  
    Sum2 = Sum2 + ( H(i,Agent_Num) * epsilon_struct(i).data );
end

Sum21 = abs(Sum2) + alpha;
SGN2 = Sum2./Sum21;

DT_i = -Observer_Gain1*epsilon_i - SGN2*diag(Upsilon_M);

end

== matlab function Cooperative_Quad_Rev01_4Agents_9/Agent #1/Decenteralized Cooperaive Controller #1/Observer q#1 ==
  data: q input; Dq_i output; tau input; H parameter; BN parameter; AN parameter; q_i input; u0 input; U_dot0_M parameter; tau_i output; N parameter; Agent_Num input; Observer_Gain parameter; n0 parameter; alpha parameter
function [Dq_i,tau_i] = fcn(q,tau,H,BN,AN,q_i,u0,U_dot0_M,N,Agent_Num,Observer_Gain,n0,alpha)

tau_i = + BN(Agent_Num,Agent_Num)*(q_i - u0);
Sum2 = zeros(n0,1);
for i=1:N
    tau_i = tau_i + ( AN(Agent_Num,i) * (q_i - q(((i-1)*n0+1):n0*i)) );  
    Sum2 = Sum2 + ( H(i,Agent_Num) * tau(((i-1)*n0+1):n0*i) );
end

Sum21 = abs(Sum2) + alpha;
SGN2 = Sum2./Sum21;

Dq_i = -Observer_Gain*tau_i - diag(SGN2)*U_dot0_M;

end

== matlab function Cooperative_Quad_Rev01_4Agents_9/Agent #2/Decenteralized Cooperaive Controller #2/Controller #2/variable change ==
  data: X input; Xd input; x_mod output; u input; xd_mod output; e_mod output; phi_d output; theta_d output
function [x_mod,xd_mod,e_mod,phi_d,theta_d] = fcn(X,Xd,u)

x_mod = X;

u0 = sqrt((u(7)^2)+(u(8)^2)+(u(9)^2));

psi_d = 0;
phi_d = asin( min(max(((sin(psi_d)*u(7) - cos(psi_d)*u(8)) / (u0+0.001)),-1),1) );
theta_d = atan( (cos(psi_d)*u(7) + sin(psi_d)*u(8)) / (u(9)+1e-3) );

PHI_d = [phi_d;theta_d;psi_d]; 

xd_mod = [Xd;PHI_d;u(1:6)];

e_mod = xd_mod - x_mod;


end

== matlab function Cooperative_Quad_Rev01_4Agents_9/Agent #1/Plant #1/MATLAB Function ==
  data: X input; u1 input; u2 input; u3 input; u4 input; t input; DX output; Kf parameter; Kt parameter; Kd parameter; Ka parameter; M parameter; J parameter; Lq parameter; g parameter
function DX = fcn(X,u1,u2,u3,u4,t,Kf,Kt,Kd,Ka,M,J,Lq,g)

F1 = Kf * u1^2;
F2 = Kf * u2^2;
F3 = Kf * u3^2;
F4 = Kf * u4^2;
 
FT = F1 + F2 + F3 + F4;

T1 = Kt * u1^2;
T2 = Kt * u2^2;
T3 = Kt * u3^2;
T4 = Kt * u4^2;

phi = X(4);
theta = X(5);
psi = X(6);

Rq = [cos(psi)*cos(theta) -sin(psi)*cos(phi)+cos(psi)*sin(theta)*sin(phi) sin(psi)*sin(phi)+cos(psi)*sin(theta)*cos(phi);
    sin(psi)*cos(theta) cos(psi)*cos(phi)+sin(psi)*sin(theta)*sin(phi) -cos(psi)*sin(phi)+sin(psi)*sin(theta)*cos(phi);
    -sin(theta) cos(theta)*sin(phi) cos(theta)*cos(phi)]; 

R_omega = [1 0 -sin(theta);
    0 cos(phi) cos(theta)*sin(phi);
    0 -sin(phi) cos(theta)*cos(phi)];

EXT_PRD = External_Product3(X(10:12),(J*X(10:12)));

DP = X(7:9);
DPHI = R_omega^(-1) * X(10:12); 
Dv = (1/M)*(Rq*[0;0;FT] - Kd*X(7:9) - M*[0;0;g]) + Rq*(1*sin(1*t))*[0;0;1];
Dw = (J^(-1))*([Lq*(F3-F1);Lq*(F4-F2);(T1-T2+T3-T4)] - Ka*X(10:12) - EXT_PRD) + (1*sin(1*t));

DX = [DP;DPHI;Dv;Dw];

end

== matlab function Cooperative_Quad_Rev01_4Agents_9/Agent #2/Decenteralized Cooperaive Controller #2/Observer T#2 ==
  data: T_struct parameter; T input; DT_i output; epsilon input; epsilon_struct parameter; H parameter; BN parameter; AN parameter; T_i input; chi input; Upsilon_M parameter; epsilon_i output; N parameter; n0 parameter; Agent_Num input; Observer_Gain1 parameter; alpha parameter
function [DT_i,epsilon_i] = fcn(T_struct,T,epsilon,epsilon_struct,H,BN,AN,T_i,chi,Upsilon_M,N,n0,...
    Agent_Num,Observer_Gain1,alpha)

T_struct(1).data = T.t1;
T_struct(2).data = T.t2;
T_struct(3).data = T.t3;
T_struct(4).data = T.t4;

epsilon_struct(1).data = epsilon.eps1;
epsilon_struct(2).data = epsilon.eps2;
epsilon_struct(3).data = epsilon.eps3;
epsilon_struct(4).data = epsilon.eps4;

epsilon_i = + BN(Agent_Num,Agent_Num)*(T_i - chi);
Sum2 = zeros(N+1,n0);
for i=1:N
    epsilon_i = epsilon_i + ( AN(Agent_Num,i) * (T_i - T_struct(i).data) );  
    Sum2 = Sum2 + ( H(i,Agent_Num) * epsilon_struct(i).data );
end

Sum21 = abs(Sum2) + alpha;
SGN2 = Sum2./Sum21;

DT_i = -Observer_Gain1*epsilon_i - SGN2*diag(Upsilon_M);

end

== matlab function Cooperative_Quad_Rev01_4Agents_9/Agent #2/Decenteralized Cooperaive Controller #2/Observer q#2 ==
  data: q input; Dq_i output; tau input; H parameter; BN parameter; AN parameter; q_i input; u0 input; U_dot0_M parameter; tau_i output; N parameter; Agent_Num input; Observer_Gain parameter; n0 parameter; alpha parameter
function [Dq_i,tau_i] = fcn(q,tau,H,BN,AN,q_i,u0,U_dot0_M,N,Agent_Num,Observer_Gain,n0,alpha)

tau_i = + BN(Agent_Num,Agent_Num)*(q_i - u0);
Sum2 = zeros(n0,1);
for i=1:N
    tau_i = tau_i + ( AN(Agent_Num,i) * (q_i - q(((i-1)*n0+1):n0*i)) );  
    Sum2 = Sum2 + ( H(i,Agent_Num) * tau(((i-1)*n0+1):n0*i) );
end

Sum21 = abs(Sum2) + alpha;
SGN2 = Sum2./Sum21;

Dq_i = -Observer_Gain*tau_i - diag(SGN2)*U_dot0_M;

end

== matlab function Cooperative_Quad_Rev01_4Agents_9/Agent #2/Plant #2/MATLAB Function ==
  data: X input; u1 input; u2 input; u3 input; u4 input; t input; DX output; Kf parameter; Kt parameter; Kd parameter; Ka parameter; M parameter; J parameter; Lq parameter; g parameter
function DX = fcn(X,u1,u2,u3,u4,t,Kf,Kt,Kd,Ka,M,J,Lq,g)

F1 = Kf * u1^2;
F2 = Kf * u2^2;
F3 = Kf * u3^2;
F4 = Kf * u4^2;
 
FT = F1 + F2 + F3 + F4;

T1 = Kt * u1^2;
T2 = Kt * u2^2;
T3 = Kt * u3^2;
T4 = Kt * u4^2;

phi = X(4);
theta = X(5);
psi = X(6);

Rq = [cos(psi)*cos(theta) -sin(psi)*cos(phi)+cos(psi)*sin(theta)*sin(phi) sin(psi)*sin(phi)+cos(psi)*sin(theta)*cos(phi);
    sin(psi)*cos(theta) cos(psi)*cos(phi)+sin(psi)*sin(theta)*sin(phi) -cos(psi)*sin(phi)+sin(psi)*sin(theta)*cos(phi);
    -sin(theta) cos(theta)*sin(phi) cos(theta)*cos(phi)]; 

R_omega = [1 0 -sin(theta);
    0 cos(phi) cos(theta)*sin(phi);
    0 -sin(phi) cos(theta)*cos(phi)];

EXT_PRD = External_Product3(X(10:12),(J*X(10:12)));

DP = X(7:9);
DPHI = R_omega^(-1) * X(10:12); 
Dv = (1/M)*(Rq*[0;0;FT] - Kd*X(7:9) - M*[0;0;g]) + Rq*(1*sin(1*t))*[0;0;1];
Dw = (J^(-1))*([Lq*(F3-F1);Lq*(F4-F2);(T1-T2+T3-T4)] - Ka*X(10:12) - EXT_PRD) + (1*sin(1*t));

DX = [DP;DPHI;Dv;Dw];

end

== matlab function Cooperative_Quad_Rev01_4Agents_9/Agent #3/Controller interpreter ==
  data: u output; U input; RM_1 parameter; n0 parameter; n parameter
function u = fcn(U,RM_1,n0,n)

y0 = sqrt((U(7)^2)+(U(8)^2)+(U(9)^2));
y1 = U(10);
y2 = U(11);
y3 = U(12);

Y = [y0;y1;y2;y3];

u = RM_1*Y;

for i=1:4
    u(i) = sqrt(abs(u(i)));
end

end

== matlab function Cooperative_Quad_Rev01_4Agents_9/Agent #3/Decenteralized Cooperaive Controller #3/Computing xd  ==
  data: q_i input; T_i input; xd output; Agent_Num input
function xd = fcn(q_i,T_i,Agent_Num)

xd = q_i + T_i(1,:)' + T_i(Agent_Num+1,:)';

end

== matlab function Cooperative_Quad_Rev01_4Agents_9/Agent #3/Decenteralized Cooperaive Controller #3/Controller #3/CARE ==
  data: P input; a_hat input; B parameter; R parameter; DP output; Q parameter
function DP = fcn(P,a_hat,B,R,Q)

DP = a_hat*P + P*a_hat' - P*B*R*B'*P + 2*Q;

end

== matlab function Cooperative_Quad_Rev01_4Agents_9/Agent #3/Decenteralized Cooperaive Controller #3/Controller #3/Differentiator/Sliding differentiator ==
  data: u output; u1 input; e input; k1 parameter; alpha1 parameter
function u = fcn(u1,e,k1,alpha1)

b=k1;

ABS = abs(e);
SGN = e ./ (ABS + alpha1);
u = u1 - b*(ABS.^0.5).*SGN;

end
